simulink subsystem "rss_SplyCurrEst"  (R2023a)
settings: Solver=VariableStepAuto  StartTime=0.0  StopTime=inf  RelTol=1e-3
undefined symbols (not defined in the file): Cdbl_iPhCurrMaxVal, Cdbl_iPhCurrPeakVal, Cdbl_iSplyCurrMaxVal, Cdbl_iSplyCurrPeakVal, Cdbl_nElecAgSpdMaxVal, Cdbl_pwrElecPwrMaxVal, Cdbl_pwrElecPwrPeakVal, Cdbl_uPhVltgMaxVal, Cdbl_uSplyVltgMaxVal, Cdbl_uSplyVltgMinVal, Cdbl_uSplyVltgPeakVal, ENM_MOTO_STATUS, Gu16_etaCtlBrd_MAP, Gu16_etaCtlBrd_MAP_ampActPhCurrAmp_X, Gu16_etaCtlBrd_MAP_nActElecSpd_Y
libraries: lib_conversion x10, simulink x1, lib_moving_average_filter x1
settings Model: DefaultTestHarness=rss_SupplyCurrentEstimation_thu  Creator=RAN2OFO  LastModifiedBy=xiaoqiang.yuan
settings OptimizationCC: ReuseModelBlockBuffer=off

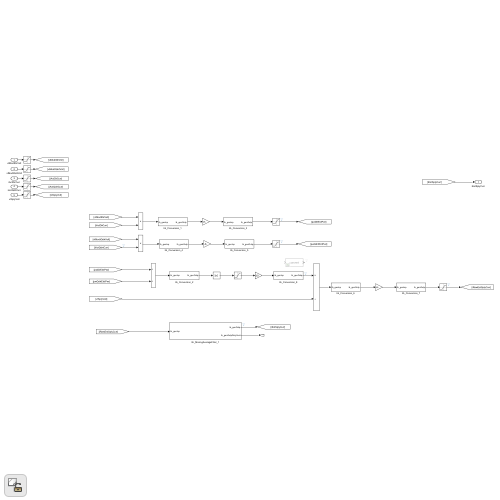
[thumbnail: Simulink's stored preview of the top-level diagram]
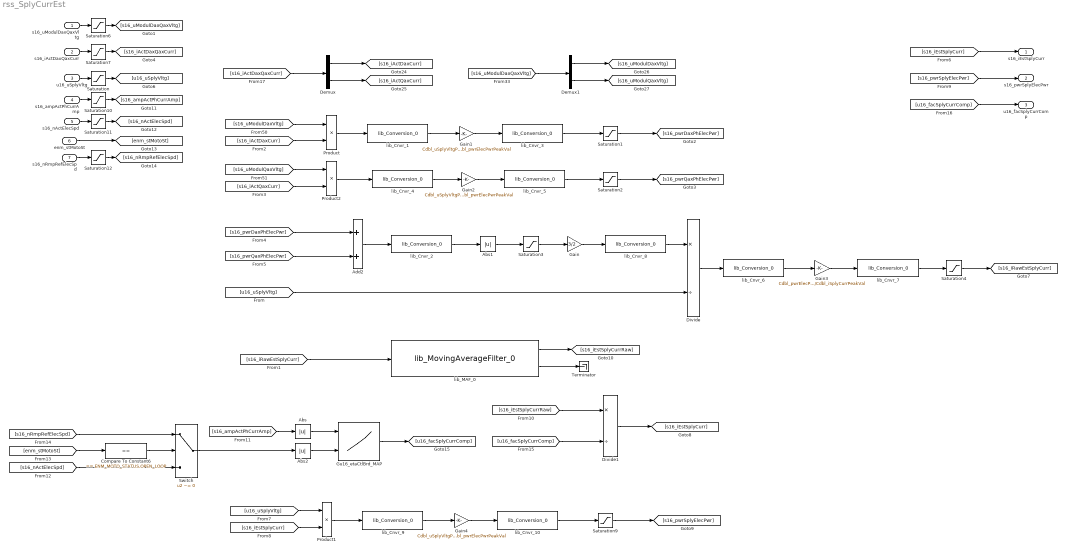
== system rss_SplyCurrEst ==
  s16_uModulDaxQaxVltg : Inport  OutDataTypeStr=dt_Standardize_s16p15b0
  s16_iActDaxQaxCurr : Inport  Port=2  OutDataTypeStr=dt_Standardize_s16p15b0
  u16_uSplyVltg : Inport  Port=3  OutDataTypeStr=dt_Standardize_u16p15b0
  s16_ampActPhCurrAmp : Inport  Port=4  OutDataTypeStr=dt_Standardize_s16p15b0
  s16_nActElecSpd : Inport  Port=5  OutDataTypeStr=dt_Standardize_s16p15b0
  enm_stMotoSt : Inport  Port=6  OutDataTypeStr=Enum: ENM_MOTO_STATUS
  s16_nRmpRefElecSpd : Inport  Port=7  OutDataTypeStr=dt_Standardize_s16p15b0
  Abs : Abs  SaturateOnIntegerOverflow=off
  Abs1 : Abs  SaturateOnIntegerOverflow=off
  Abs2 : Abs  SaturateOnIntegerOverflow=off
  Add2 : Sum  OutDataTypeStr=Inherit: Inherit via back propagation
  Compare To Constant6 : simulink/Logic and Bit Operations/Compare To Constant  relop===  const=ENM_MOTO_STATUS.OPEN_LOOP  OutDataTypeStr=boolean
  Demux : Demux  Outputs=2
  Demux1 : Demux  Outputs=2
  Divide : Product  Inputs=*/  OutDataTypeStr=Inherit: Inherit via back propagation  RndMeth=Simplest
  Divide1 : Product  Inputs=*/  OutDataTypeStr=Inherit: Same as first input
  Gain : Gain  Gain=3/2  OutDataTypeStr=Inherit: Inherit via back propagation  RndMeth=Simplest
  Gain1 : Gain  Gain=Cdbl_uSplyVltgPeakVal*Cdbl_iPhCurrPeakVal/Cdbl_pwrElecPwrPeakVal  OutDataTypeStr=Inherit: Inherit via back propagation  RndMeth=Simplest
  Gain2 : Gain  Gain=Cdbl_uSplyVltgPeakVal*Cdbl_iPhCurrPeakVal/Cdbl_pwrElecPwrPeakVal  OutDataTypeStr=Inherit: Inherit via back propagation  RndMeth=Simplest
  Gain3 : Gain  Gain=Cdbl_pwrElecPwrPeakVal/Cdbl_uSplyVltgPeakVal/Cdbl_iSplyCurrPeakVal  OutDataTypeStr=Inherit: Inherit via back propagation  RndMeth=Simplest
  Gain4 : Gain  Gain=Cdbl_uSplyVltgPeakVal*Cdbl_iSplyCurrPeakVal/Cdbl_pwrElecPwrPeakVal  OutDataTypeStr=Inherit: Inherit via back propagation  RndMeth=Simplest
  Gu16_etaCtlBrd_MAP : Lookup_n-D  BreakpointsForDimension1=Gu16_etaCtlBrd_MAP_ampActPhCurrAmp_X  BreakpointsForDimension2=Gu16_etaCtlBrd_MAP_nActElecSpd_Y  Table=Gu16_etaCtlBrd_MAP  ExtrapMethod=Clip  InternalRulePriority=Speed  OutDataTypeStr=Inherit: Inherit from 'Table data'  RndMeth=Simplest
      settings: InputPortMap=u0,u1
  Product : Product  OutDataTypeStr=Inherit: Inherit via back propagation
  Product1 : Product  OutDataTypeStr=Inherit: Inherit via back propagation
  Product2 : Product  OutDataTypeStr=Inherit: Inherit via back propagation
  Saturation : Saturate  UpperLimit=Cdbl_uSplyVltgMaxVal  LowerLimit=Cdbl_uSplyVltgMinVal
  Saturation1 : Saturate  UpperLimit=Cdbl_pwrElecPwrMaxVal  LowerLimit=-Cdbl_pwrElecPwrMaxVal
  Saturation10 : Saturate  UpperLimit=Cdbl_iPhCurrMaxVal  LowerLimit=-Cdbl_iPhCurrMaxVal
  Saturation11 : Saturate  UpperLimit=Cdbl_nElecAgSpdMaxVal  LowerLimit=-Cdbl_nElecAgSpdMaxVal
  Saturation12 : Saturate  UpperLimit=Cdbl_nElecAgSpdMaxVal  LowerLimit=-Cdbl_nElecAgSpdMaxVal
  Saturation2 : Saturate  UpperLimit=Cdbl_pwrElecPwrMaxVal  LowerLimit=-Cdbl_pwrElecPwrMaxVal
  Saturation3 : Saturate  UpperLimit=Cdbl_pwrElecPwrMaxVal  LowerLimit=0
  Saturation4 : Saturate  UpperLimit=Cdbl_iSplyCurrMaxVal  LowerLimit=0
  Saturation6 : Saturate  UpperLimit=Cdbl_uPhVltgMaxVal  LowerLimit=-Cdbl_uPhVltgMaxVal
  Saturation7 : Saturate  UpperLimit=Cdbl_iPhCurrMaxVal  LowerLimit=-Cdbl_iPhCurrMaxVal
  Saturation9 : Saturate  UpperLimit=Cdbl_pwrElecPwrMaxVal  LowerLimit=-Cdbl_pwrElecPwrMaxVal
  Switch : Switch  Criteria=u2 ~= 0  SaturateOnIntegerOverflow=off  InputSameDT=off
  Terminator : Terminator
  lib_Cnvr_1 : lib_conversion/lib_Conversion_0  lb_parDataType=fixdt(1,16)  lb_parOutpMaxVal=Cdbl_iPhCurrMaxVal*Cdbl_uPhVltgMaxVal  lb_parOutpMinVal=[]  lb_parSatFlag=off
  lib_Cnvr_{3,5,7,10} (4 alike) : lib_conversion/lib_Conversion_0  lb_parDataType=dt_Standardize_s16p15b0  lb_parOutpMaxVal=[]  lb_parOutpMinVal=[]  lb_parSatFlag=off
  lib_Cnvr_2 : lib_conversion/lib_Conversion_0  lb_parDataType=fixdt(1,16)  lb_parOutpMaxVal=2*Cdbl_pwrElecPwrMaxVal  lb_parOutpMinVal=-2*Cdbl_pwrElecPwrMaxVal  lb_parSatFlag=off
  lib_Cnvr_4 : lib_conversion/lib_Conversion_0  lb_parDataType=fixdt(1,16)  lb_parOutpMaxVal=Cdbl_iPhCurrMaxVal*Cdbl_uPhVltgMaxVal  lb_parOutpMinVal=[]  lb_parSatFlag=off
  lib_Cnvr_6 : lib_conversion/lib_Conversion_0  lb_parDataType=fixdt(0,16)  lb_parOutpMaxVal=3/2*Cdbl_pwrElecPwrMaxVal/Cdbl_uSplyVltgMinVal  lb_parOutpMinVal=[]  lb_parSatFlag=off
  lib_Cnvr_8 : lib_conversion/lib_Conversion_0  lb_parDataType=fixdt(0,16)  lb_parOutpMaxVal=3/2*Cdbl_pwrElecPwrMaxVal  lb_parOutpMinVal=[]  lb_parSatFlag=off
  lib_Cnvr_9 : lib_conversion/lib_Conversion_0  lb_parDataType=fixdt(1,16)  lb_parOutpMaxVal=Cdbl_iSplyCurrMaxVal*Cdbl_uSplyVltgMaxVal  lb_parOutpMinVal=[]  lb_parSatFlag=off
  lib_MAF_0 : lib_moving_average_filter/lib_MovingAverageFilter_0  lb_parSampNum=Cdbl_numSplyCurrMAFSmpNum  lb_parInpSmtnDataType=fixdt(1,32,2^-19,0)
  s16_iEstSplyCurr : Outport  OutDataTypeStr=dt_Standardize_s16p15b0
  s16_pwrSplyElecPwr : Outport  Port=2  OutDataTypeStr=dt_Standardize_s16p15b0
  u16_facSplyCurrComp : Outport  Port=3  OutDataTypeStr=dt_Standardize_u16p15b0
  wires:
  [s16_iRawEstSplyCurr] -> lib_MAF_0/1
  s16_iActDaxQaxCurr/1 -> Saturation7/1
  [u16_uSplyVltg] -> Divide/2
  Divide/1 -> lib_Cnvr_6/1
  lib_Cnvr_2/1 -> Abs1/1
  Product/1 -> lib_Cnvr_1/1
  Add2/1 -> lib_Cnvr_2/1
  Gain/1 -> lib_Cnvr_8/1
  s16_uModulDaxQaxVltg/1 -> Saturation6/1
  [s16_uModulDaxVltg] -> Product/1
  [s16_iActDaxCurr] -> Product/2
  Product2/1 -> lib_Cnvr_4/1
  [s16_uModulQaxVltg] -> Product2/1
  [s16_iActQaxCurr] -> Product2/2
  lib_Cnvr_1/1 -> Gain1/1
  [s16_pwrQaxPhElecPwr] -> Add2/2
  [s16_pwrDaxPhElecPwr] -> Add2/1
  u16_uSplyVltg/1 -> Saturation/1
  Abs1/1 -> Saturation3/1
  lib_Cnvr_8/1 -> Divide/1
  Saturation4/1 -> [s16_iRawEstSplyCurr]
  lib_MAF_0/2 -> Terminator/1
  lib_MAF_0/1 -> [s16_iEstSplyCurrRaw]
  [s16_iEstSplyCurr] -> s16_iEstSplyCurr/1
  Saturation1/1 -> [s16_pwrDaxPhElecPwr]
  Saturation2/1 -> [s16_pwrQaxPhElecPwr]
  Saturation3/1 -> Gain/1
  Saturation/1 -> [u16_uSplyVltg]
  Saturation6/1 -> [s16_uModulDaxQaxVltg]
  Saturation7/1 -> [s16_iActDaxQaxCurr]
  Gain1/1 -> lib_Cnvr_3/1
  lib_Cnvr_3/1 -> Saturation1/1
  Gain2/1 -> lib_Cnvr_5/1
  lib_Cnvr_5/1 -> Saturation2/1
  lib_Cnvr_4/1 -> Gain2/1
  Gain3/1 -> lib_Cnvr_7/1
  lib_Cnvr_6/1 -> Gain3/1
  lib_Cnvr_7/1 -> Saturation4/1
  Gain4/1 -> lib_Cnvr_10/1
  Product1/1 -> lib_Cnvr_9/1
  lib_Cnvr_9/1 -> Gain4/1
  lib_Cnvr_10/1 -> Saturation9/1
  [u16_uSplyVltg] -> Product1/1
  [s16_iEstSplyCurr] -> Product1/2
  Saturation9/1 -> [s16_pwrSplyElecPwr]
  [s16_pwrSplyElecPwr] -> s16_pwrSplyElecPwr/1
  [s16_iEstSplyCurrRaw] -> Divide1/1
  Divide1/1 -> [s16_iEstSplyCurr]
  s16_ampActPhCurrAmp/1 -> Saturation10/1
  Saturation10/1 -> [s16_ampActPhCurrAmp]
  s16_nActElecSpd/1 -> Saturation11/1
  Saturation11/1 -> [s16_nActElecSpd]
  [s16_ampActPhCurrAmp] -> Abs/1
  Switch/1 -> Abs2/1
  Abs/1 -> Gu16_etaCtlBrd_MAP/1
  Abs2/1 -> Gu16_etaCtlBrd_MAP/2
  enm_stMotoSt/1 -> [enm_stMotoSt]
  [enm_stMotoSt] -> Compare To Constant6/1
  Saturation12/1 -> [s16_nRmpRefElecSpd]
  s16_nRmpRefElecSpd/1 -> Saturation12/1
  Compare To Constant6/1 -> Switch/2
  [s16_nRmpRefElecSpd] -> Switch/1
  [s16_nActElecSpd] -> Switch/3
  Gu16_etaCtlBrd_MAP/1 -> [u16_facSplyCurrComp]
  [u16_facSplyCurrComp] -> Divide1/2
  [u16_facSplyCurrComp] -> u16_facSplyCurrComp/1
  Demux/2 -> [s16_iActQaxCurr]
  [s16_iActDaxQaxCurr] -> Demux/1
  Demux/1 -> [s16_iActDaxCurr]
  [s16_uModulDaxQaxVltg] -> Demux1/1
  Demux1/1 -> [s16_uModulDaxVltg]
  Demux1/2 -> [s16_uModulQaxVltg]
